simulink model "apartado2_2_1"  (R2019b)
settings: Solver=VariableStepAuto  StartTime=0.0  StopTime=500  RelTol=1e-3
settings Model: Creator=pablo  LastModifiedBy=pablo

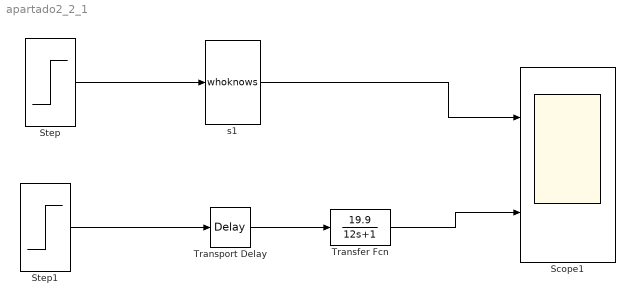
== system apartado2_2_1 ==
  Scope1 : Scope  NumInputPorts=2
  Step : Step  SampleTime=0
  Step1 : Step  SampleTime=0
  Transfer Fcn : TransferFcn  Numerator=[19.9]  Denominator=[12 1]
  Transport Delay : TransportDelay  DelayTime=2
  s1 : M-S-Function  FunctionName=whoknows  Parameters=L, P1, P2, T, R  mask{L=7, P1=0, P2=7, T=1, R=0}
      mask prompts: L "Laboratorio"; P1 "Primer digito del Puesto"; P2 "Segundo digito del Puesto"; T "Tipo de Planta"; R "Ruido"
      mask Display: disp('Sistema')
  wires:
  Transport Delay/1 -> Transfer Fcn/1
  Step1/1 -> Transport Delay/1
  Transfer Fcn/1 -> Scope1/2
  Step/1 -> s1/1
  s1/1 -> Scope1/1
